simulink model "model"  (R2014a)
(part 5 of 5)

  T_240018999__/RConn1 -- L_240018999/LConn1
  T_240018999__/RConn2 -- L_240018999/LConn2
  L_240018999/LConn3 -- T_240018999__/RConn3 -- bus449/LConn1
  T_158349339_220000_Подстанция_220_кВ_Космос/RConn1 -- L_158349339/LConn1
  T_158349339_220000_Подстанция_220_кВ_Космос/RConn2 -- L_158349339/LConn2
  L_158349339/LConn3 -- T_158349339_220000_Подстанция_220_кВ_Космос/RConn3 -- bus450/LConn1
  T_306106528__Екатериновка_газовая/RConn1 -- L_306106528/LConn1
  T_306106528__Екатериновка_газовая/RConn2 -- L_306106528/LConn2
  L_306106528/LConn3 -- T_306106528__Екатериновка_газовая/RConn3 -- bus451/LConn1
  T_328463572__/RConn1 -- L_328463572/LConn1
  T_328463572__/RConn2 -- L_328463572/LConn2
  L_328463572/LConn3 -- T_328463572__/RConn3 -- bus452/LConn1
  T_224261932__Аткарская/RConn1 -- L_224261932/LConn1
  T_224261932__Аткарская/RConn2 -- L_224261932/LConn2
  L_224261932/LConn3 -- T_224261932__Аткарская/RConn3 -- bus453/LConn1
  T_327226015_220000_Починковская_2/RConn1 -- L_327226015/LConn1
  T_327226015_220000_Починковская_2/RConn2 -- L_327226015/LConn2
  L_327226015/LConn3 -- T_327226015_220000_Починковская_2/RConn3 -- bus454/LConn1
  T_103735794_220000_Центролит/RConn1 -- L_103735794/LConn1
  T_103735794_220000_Центролит/RConn2 -- L_103735794/LConn2
  L_103735794/LConn3 -- T_103735794_220000_Центролит/RConn3 -- bus455/LConn1
  T_48949159_220000;35000_/RConn1 -- L_48949159/LConn1
  T_48949159_220000;35000_/RConn2 -- L_48949159/LConn2
  L_48949159/LConn3 -- T_48949159_220000;35000_/RConn3 -- bus456/LConn1
  T_51711046_220000;110000;fixme_/RConn1 -- L_51711046/LConn1
  T_51711046_220000;110000;fixme_/RConn2 -- L_51711046/LConn2
  L_51711046/LConn3 -- T_51711046_220000;110000;fixme_/RConn3 -- bus457/LConn1
  T_276080500_220000_Комсомольская/RConn1 -- L_276080500/LConn1
  T_276080500_220000_Комсомольская/RConn2 -- L_276080500/LConn2
  L_276080500/LConn3 -- T_276080500_220000_Комсомольская/RConn3 -- bus458/LConn1
  T_96826924_220000;110000;10000_ПС_220_кВ_Новотроицкая/RConn1 -- L_96826924/LConn1
  T_96826924_220000;110000;10000_ПС_220_кВ_Новотроицкая/RConn2 -- L_96826924/LConn2
  L_96826924/LConn3 -- T_96826924_220000;110000;10000_ПС_220_кВ_Новотроицкая/RConn3 -- bus459/LConn1
  T_137376045__/RConn1 -- L_137376045/LConn1
  T_137376045__/RConn2 -- L_137376045/LConn2
  L_137376045/LConn3 -- T_137376045__/RConn3 -- bus460/LConn1
  T_132783542_220000_ПС_Волжская/RConn1 -- L_132783542/LConn1
  T_132783542_220000_ПС_Волжская/RConn2 -- L_132783542/LConn2
  L_132783542/LConn3 -- T_132783542_220000_ПС_Волжская/RConn3 -- bus461/LConn1
  T_327226025_220000_Починковская_1/RConn1 -- L_327226025/LConn1
  T_327226025_220000_Починковская_1/RConn2 -- L_327226025/LConn2
  L_327226025/LConn3 -- T_327226025_220000_Починковская_1/RConn3 -- bus462/LConn1
  T_96563667__/RConn1 -- L_96563667/LConn1
  T_96563667__/RConn2 -- L_96563667/LConn2
  L_96563667/LConn3 -- T_96563667__/RConn3 -- bus463/LConn1
  T_95488527_220000;110000;35000;6000_ПС_Абдрахманово/RConn1 -- L_95488527/LConn1
  T_95488527_220000;110000;35000;6000_ПС_Абдрахманово/RConn2 -- L_95488527/LConn2
  L_95488527/LConn3 -- T_95488527_220000;110000;35000;6000_ПС_Абдрахманово/RConn3 -- bus464/LConn1
  T_95488500__ПС_Письмянка/RConn1 -- L_95488500/LConn1
  T_95488500__ПС_Письмянка/RConn2 -- L_95488500/LConn2
  L_95488500/LConn3 -- T_95488500__ПС_Письмянка/RConn3 -- bus465/LConn1
  T_274213600_220000_ПС_Студенец/RConn1 -- L_274213600/LConn1
  T_274213600_220000_ПС_Студенец/RConn2 -- L_274213600/LConn2
  L_274213600/LConn3 -- T_274213600_220000_ПС_Студенец/RConn3 -- bus466/LConn1
  T_82458858_220000_ОРУ_220_кВ/RConn1 -- L_82458858/LConn1
  T_82458858_220000_ОРУ_220_кВ/RConn2 -- L_82458858/LConn2
  L_82458858/LConn3 -- T_82458858_220000_ОРУ_220_кВ/RConn3 -- bus467/LConn1
  T_110601218_500000_/RConn1 -- L_110601218/LConn1
  T_110601218_500000_/RConn2 -- L_110601218/LConn2
  L_110601218/LConn3 -- T_110601218_500000_/RConn3 -- bus468/LConn1
  T_131490223__ПС_Вешкайма/RConn1 -- L_131490223/LConn1
  T_131490223__ПС_Вешкайма/RConn2 -- L_131490223/LConn2
  L_131490223/LConn3 -- T_131490223__ПС_Вешкайма/RConn3 -- bus469/LConn1
  T_136586702_500000;220000;110000_ПС_Азот/RConn1 -- L_136586702/LConn1
  T_136586702_500000;220000;110000_ПС_Азот/RConn2 -- L_136586702/LConn2
  L_136586702/LConn3 -- T_136586702_500000;220000;110000_ПС_Азот/RConn3 -- bus470/LConn1
  T_219655813_500000;220000;110000_ПС_Буйская/RConn1 -- L_219655813/LConn1
  T_219655813_500000;220000;110000_ПС_Буйская/RConn2 -- L_219655813/LConn2
  L_219655813/LConn3 -- T_219655813_500000;220000;110000_ПС_Буйская/RConn3 -- bus471/LConn1
  T_53015400_500000_ПС_Калино/RConn1 -- L_53015400/LConn1
  T_53015400_500000_ПС_Калино/RConn2 -- L_53015400/LConn2
  L_53015400/LConn3 -- T_53015400_500000_ПС_Калино/RConn3 -- bus472/LConn1
  T_376942192__/RConn1 -- L_376942192/LConn1
  T_376942192__/RConn2 -- L_376942192/LConn2
  L_376942192/LConn3 -- T_376942192__/RConn3 -- bus473/LConn1
  T_114285735_500000;220000;10000_ПС_Уфимская/RConn1 -- L_114285735/LConn1
  T_114285735_500000;220000;10000_ПС_Уфимская/RConn2 -- L_114285735/LConn2
  L_114285735/LConn3 -- T_114285735_500000;220000;10000_ПС_Уфимская/RConn3 -- bus474/LConn1
  T_92325642_500000_Радуга/RConn1 -- L_92325642/LConn1
  T_92325642_500000_Радуга/RConn2 -- L_92325642/LConn2
  L_92325642/LConn3 -- T_92325642_500000_Радуга/RConn3 -- bus475/LConn1
  T_150285837_500000;220000;110000_ПС_Бекетово/RConn1 -- L_150285837/LConn1
  T_150285837_500000;220000;110000_ПС_Бекетово/RConn2 -- L_150285837/LConn2
  L_150285837/LConn3 -- T_150285837_500000;220000;110000_ПС_Бекетово/RConn3 -- bus476/LConn1
  "T_88028486_500000_ПС_500_кВ_\"Бугульма\""/RConn1 -- L_88028486/LConn1
  "T_88028486_500000_ПС_500_кВ_\"Бугульма\""/RConn2 -- L_88028486/LConn2
  L_88028486/LConn3 -- "T_88028486_500000_ПС_500_кВ_\"Бугульма\""/RConn3 -- bus477/LConn1
  "T_99190583_500000;220000;110000;fixme_\"Смеловская\"_500_кВ"/RConn1 -- L_99190583/LConn1
  "T_99190583_500000;220000;110000;fixme_\"Смеловская\"_500_кВ"/RConn2 -- L_99190583/LConn2
  L_99190583/LConn3 -- "T_99190583_500000;220000;110000;fixme_\"Смеловская\"_500_кВ"/RConn3 -- bus478/LConn1
  T_131508245_500000_ПС_Ключики/RConn1 -- L_131508245/LConn1
  T_131508245_500000_ПС_Ключики/RConn2 -- L_131508245/LConn2
  L_131508245/LConn3 -- T_131508245_500000_ПС_Ключики/RConn3 -- bus479/LConn1
  T_193513250__/RConn1 -- L_193513250/LConn1
  T_193513250__/RConn2 -- L_193513250/LConn2
  L_193513250/LConn3 -- T_193513250__/RConn3 -- bus480/LConn1
  T_219112646__/RConn1 -- L_219112646/LConn1
  T_219112646__/RConn2 -- L_219112646/LConn2
  L_219112646/LConn3 -- T_219112646__/RConn3 -- bus481/LConn1
  T_363144177__ОРУ_500_кВ_ИрГРЭС___1/RConn1 -- L_363144177/LConn1
  T_363144177__ОРУ_500_кВ_ИрГРЭС___1/RConn2 -- L_363144177/LConn2
  L_363144177/LConn3 -- T_363144177__ОРУ_500_кВ_ИрГРЭС___1/RConn3 -- bus482/LConn1
  T_90273320__Курдюм/RConn1 -- L_90273320/LConn1
  T_90273320__Курдюм/RConn2 -- L_90273320/LConn2
  L_90273320/LConn3 -- T_90273320__Курдюм/RConn3 -- bus483/LConn1
  T_82967790__ПС_Пенза_2/RConn1 -- L_82967790/LConn1
  T_82967790__ПС_Пенза_2/RConn2 -- L_82967790/LConn2
  L_82967790/LConn3 -- T_82967790__ПС_Пенза_2/RConn3 -- bus484/LConn1
  T_227835712_500000;220000_ПС_500_кВ_Красноармейская/RConn1 -- L_227835712/LConn1
  T_227835712_500000;220000_ПС_500_кВ_Красноармейская/RConn2 -- L_227835712/LConn2
  L_227835712/LConn3 -- T_227835712_500000;220000_ПС_500_кВ_Красноармейская/RConn3 -- bus485/LConn1
  T_229649869_500000_ПС_500_кВ_Удмуртская/RConn1 -- L_229649869/LConn1
  T_229649869_500000_ПС_500_кВ_Удмуртская/RConn2 -- L_229649869/LConn2
  L_229649869/LConn3 -- T_229649869_500000_ПС_500_кВ_Удмуртская/RConn3 -- bus486/LConn1
  T_82459105_500000_ОРУ_500_кВ/RConn1 -- L_82459105/LConn1
  T_82459105_500000_ОРУ_500_кВ/RConn2 -- L_82459105/LConn2
  L_82459105/LConn3 -- T_82459105_500000_ОРУ_500_кВ/RConn3 -- bus487/LConn1
  T_169556579__ПC_Приваловская_500_кВ/RConn1 -- L_169556579/LConn1
  T_169556579__ПC_Приваловская_500_кВ/RConn2 -- L_169556579/LConn2
  L_169556579/LConn3 -- T_169556579__ПC_Приваловская_500_кВ/RConn3 -- bus488/LConn1
  T_113767652_500000_ПС_Кропачево/RConn1 -- L_113767652/LConn1
  T_113767652_500000_ПС_Кропачево/RConn2 -- L_113767652/LConn2
  L_113767652/LConn3 -- T_113767652_500000_ПС_Кропачево/RConn3 -- bus489/LConn1
